simulink subsystem "stateMachine"  (R2020b)
settings: Solver=VariableStepAuto  StartTime=0.0  StopTime=10.0  RelTol=1e-3
settings Model: Creator=galli  LastModifiedBy=galli

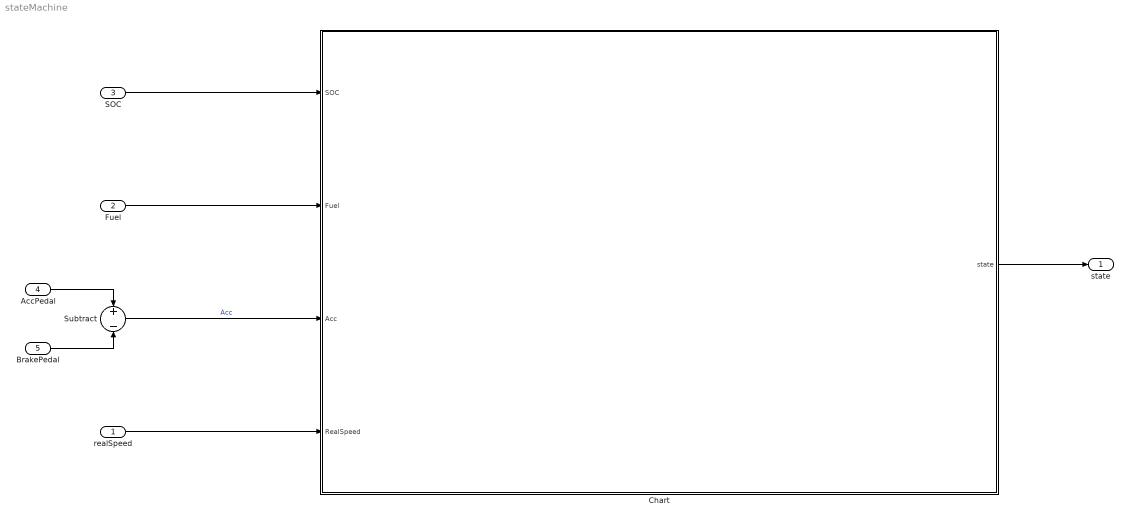
== system stateMachine ==
  realSpeed : Inport
  Fuel : Inport  Port=2
  SOC : Inport  Port=3
  AccPedal : Inport  Port=4
  BrakePedal : Inport  Port=5
  Chart : Stateflow chart  TreatAsAtomicUnit=on
  Subtract : Sum  Inputs=+-
  state : Outport
  wires:
  AccPedal/1 -> Subtract/1
  Subtract/1 -> Chart/3(Acc)  "Acc"
  BrakePedal/1 -> Subtract/2
  realSpeed/1 -> Chart/4(RealSpeed)
  SOC/1 -> Chart/1(SOC)
  Fuel/1 -> Chart/2(Fuel)
  Chart/1(state) -> state/1

== stateflow chart stateMachine/Chart ==
  state Dead
    %Dead state. It occurs when there is no fuel in the tank and not charge in the battery
    state = 0;
  state NoCharge
    %occurs when the battery SOC is under a treshold. The car switch full ICE
    state=1;
  state ED
    %Electric drive. Occurs when forced by the city zone of under a reference speed
    %imponi v<vedmax se non vi è benzina
    state=2;
  state Combined
    %)(Hybrid drive) over a certain spped both the engine will collaborate to give the required torque
    %IMPONI V<VEDmin se finisce il carburante prima di andare in ED
    state=3;
  state Rigenerative_Braking
    %you will go in that state every time you brake. So the acceleration will be lower than zero.
    %this will so charge the battery til to reach the SOCmax that will limit my case
    state=4;
  Rigenerative_Braking -> Dead [order 2] : [(SOC < SOCmin+SOCth) && (Fuel<fuelMin+fuelHys) ]
  (default) -> Dead
  Dead -> Rigenerative_Braking [order 1] : [Acc<0]
  Dead -> NoCharge [order 4] : [ (Fuel>fuelMin+fuelHys)]
  Dead -> ED [order 3] : [(SOC > SOCmin+SOCth)]
  NoCharge -> Dead [order 2] : [(Fuel<fuelMin+fuelHys) && (SOC <=SOCmin+SOCth)]
  ED -> Dead [order 2] : [(SOC<SOCmin+SOCth) && (Fuel<fuelMin+fuelHys) ]
  Combined -> Dead [order 2] : [(Fuel<fuelMin+fuelHys) && (SOC <=SOCmin+SOCth)]
  Dead -> Combined [order 2] : [(SOC > SOCmin+SOCth) && (Acc>maxAccICE || Acc>maxAccMGU) && (Fuel>fuelMin+fuelHys)]
  ED -> NoCharge [order 3] : [(Fuel>fuelMin+fuelHys) && (SOC <=SOCmin+SOCth)]
  Rigenerative_Braking -> NoCharge [order 4] : [ (Fuel>fuelMin+fuelHys)&& (SOC < SOCmin+SOCth)]
  NoCharge -> ED [order 3] : [((SOC > SOCmin+SOCth) && (RealSpeed < SpeedEDmax)) || ((Fuel<fuelMin+fuelHys) && (SOC >SOCmin+SOCth))]
  NoCharge -> Rigenerative_Braking [order 1] : [Acc<0]
  Combined -> NoCharge [order 4] : [(SOC <= SOCmin + SOCth)&&(Fuel>fuelMin+fuelHys)]
  NoCharge -> Combined [order 4] : [(SOC > SOCmin+SOCth) && (Fuel>fuelMin+fuelHys) &&Acc>maxAccICE]
  ED -> Combined [order 4] : [((RealSpeed>=SpeedEDmax)&& (Fuel>fuelMin+fuelHys))|| ((Fuel>fuelMin+fuelHys)  && Acc>maxAccMGU)]
  Combined -> ED [order 3] : [(RealSpeed<SpeedEDmax)&& (SOC >SOCmin+SOCth)&&Acc<maxAccMGU]
  Rigenerative_Braking -> ED [order 3] : [(SOC > SOCmin+SOCth) && (RealSpeed<SpeedEDmax)]
  ED -> Rigenerative_Braking [order 1] : [Acc<0]
  Combined -> Rigenerative_Braking [order 1] : [Acc < 0]
  Rigenerative_Braking -> Combined [order 5] : [(SOC > SOCmin+SOCth) && (RealSpeed>SpeedEDmax) && (Fuel>fuelMin+fuelHys)]
  Rigenerative_Braking -> Rigenerative_Braking [order 1] : [Acc<0]
  data: SOC input; Fuel input; Acc input; RealSpeed input; state output; SpeedEDmax constant double =45; fuelMin constant double =0.33; SOCth constant double =5; SOCmin constant double =10; fuelHys constant double =0.17; maxAccICE constant double =TrqICMax/TrqMax; maxAccMGU constant double =TrqMGUMax/TrqMax
